simulink model "inv_pend_sim_with_MPC_nonlin"  (R2016a)
settings: Solver=ode45  StartTime=0.0  StopTime=tf  RelTol=1e-3
values from neighbouring files (symbols this model uses):
  K = zeros(1,4)    [inv_pend.m]
  P = [M,m,L,b,J,g]    [inv_pend.m]
  T = [0,0;0,-m*g*L*cos(th_e)]    [finaltry.m]    (also in inv_pend.m = 0.1)
  Ts = T    (= 0.1)    [inv_pend.m]
  x0 = [0;th_e - 5*pi/180;0;0]    [inv_pend.m]
undefined symbols (not defined in the file or in its folder): finaltry
settings Model: Creator=nashal  LastModifiedBy=nash
settings DataIOCC: LimitDataPoints=on  SaveFormat=Array
settings HardwareCC: ProdBitPerPointer=32  ProdLargestAtomicFloat=None  ProdIntDivRoundTo=Undefined  ProdEndianess=Unspecified  ProdWordSize=32  ProdHWDeviceType=32-bit Generic
settings ModelReferenceCC: PropagateSignalLabelsOutOfModel=off
settings ConfigComp: CovModelRefEnable=Off

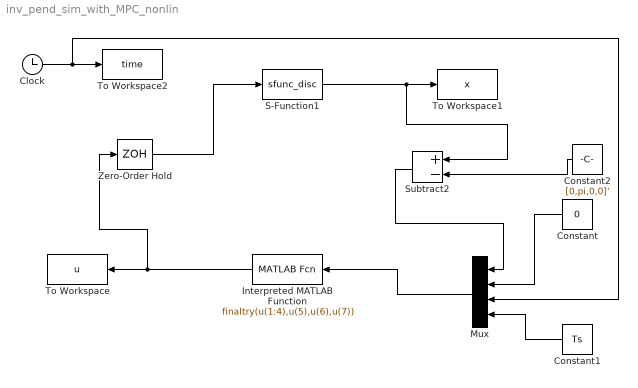
== system inv_pend_sim_with_MPC_nonlin ==
  Clock : Clock
  Constant : Constant  Value=0  SampleTime=T
  Constant1 : Constant  Value=Ts  SampleTime=T
  Constant2 : Constant  Value=[0,pi,0,0]'  SampleTime=T
  Interpreted MATLAB Function : MATLABFcn  MATLABFcn=finaltry(u(1:4),u(5),u(6),u(7))
  Mux : Mux
  S-Function1 : S-Function  FunctionName=sfunc_disc  Parameters=x0,P,K  SFunctionDeploymentMode=off  EnableBusSupport=off
  Subtract2 : Sum  Inputs=+-
  To Workspace : ToWorkspace  VariableName=u  SampleTime=T
  To Workspace1 : ToWorkspace  VariableName=x  SampleTime=T
  To Workspace2 : ToWorkspace  VariableName=time  SampleTime=T
  Zero-Order Hold : ZeroOrderHold  SampleTime=T
  wires:
  Clock/1 -> Mux/3, To Workspace2/1
  Interpreted MATLAB Function/1 -> Zero-Order Hold/1, To Workspace/1
  Mux/1 -> Interpreted MATLAB Function/1
  Constant/1 -> Mux/2
  S-Function1/1 -> Subtract2/1, To Workspace1/1
  Zero-Order Hold/1 -> S-Function1/1
  Constant2/1 -> Subtract2/2
  Subtract2/1 -> Mux/1
  Constant1/1 -> Mux/4
